simulink model "motormodelsimulink"  (R2015a)
settings: Solver=ode45  StartTime=0.0  StopTime=10  RelTol=1e-3
values from neighbouring files (symbols this model uses):
  Ke = 1.89e-3    (= 0.00189)    [motormodelscriptsimulink.m]
  Kt = 0.0016    [motormodelscriptsimulink.m]
  L = 119.26e-6    (= 0.00011926)    [motormodelscriptsimulink.m]
  R = 0.178    [motormodelscriptsimulink.m]
undefined symbols (not defined in the file or in its folder): B, J
settings Model: Creator=Amalie  LastModifiedBy=Amalie

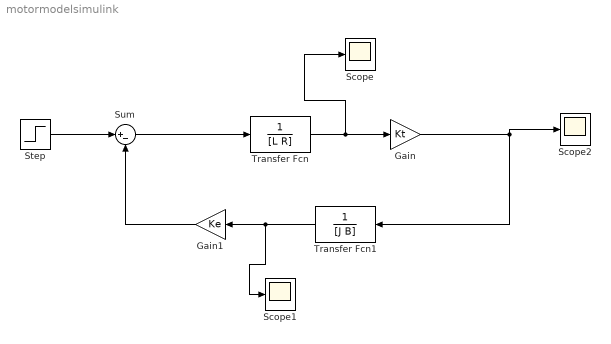
== system motormodelsimulink ==
  Gain : Gain  Gain=Kt
  Gain1 : Gain  Gain=Ke
  Scope : Scope
  Scope1 : Scope
  Scope2 : Scope
      settings: SaveName=ScopeData2
  Step : Step  After=7  SampleTime=0.01
  Sum : Sum  Inputs=|+-
  Transfer Fcn : TransferFcn  Denominator=[L R]
  Transfer Fcn1 : TransferFcn  Denominator=[J B]
  wires:
  Transfer Fcn/1 -> Scope/1, Gain/1
  Gain/1 -> Transfer Fcn1/1, Scope2/1
  Transfer Fcn1/1 -> Scope1/1, Gain1/1
  Sum/1 -> Transfer Fcn/1
  Gain1/1 -> Sum/2
  Step/1 -> Sum/1
